simulink model "Model_simulink_no_Torque"  (R2017a)
settings: Solver=ode3  StartTime=0.0  StopTime=Tend  FixedStep=0.0006  RelTol=1e-3
values from neighbouring files (symbols this model uses):
  In = 130.7    [Skrypt_do_schematu.m]
  J = Js+Jmr    (= 5.82)    [Skrypt_do_schematu.m]
  Kp = 0.15*Un    (= 66)    [Skrypt_do_schematu.m]
  Kt = 10/(1.2*wn)    (= 0.0548810148593)    [Skrypt_do_schematu.m]
  Kw = J/(2*Kt*kz*Beta*psi)    [Skrypt_do_schematu.m]
  Lambda = 2    [Skrypt_do_schematu.m]
  m = T1    [Skrypt_do_schematu.m]
  Mn = psi * In    (= 350.156554572)    [Skrypt_do_schematu.m]
  psi = (Un-(Rt*In))/wn    (= 2.67908610996)    [Skrypt_do_schematu.m]
  Rt = 0.254    [Skrypt_do_schematu.m]
  T = Lt/Rt    (= 0.00641732283465)    [Skrypt_do_schematu.m]
  TR = 4*Beta    (= 0.16)    [Skrypt_do_schematu.m]
  Un = 440    [Skrypt_do_schematu.m]
  Uz0 = (Lambda*In)*((Y*B1)/(B1-Beta))    [Skrypt_do_schematu.m]
  V = (Beta*(Y*Kp*B))/((B1-Beta)*Rt)    [Skrypt_do_schematu.m]
  wn = (2*pi*n)/60    (= 151.843644924)    [Skrypt_do_schematu.m]
  Y = 7.8/(2.5*In)    (= 0.0238714613619)    [Skrypt_do_schematu.m]
settings Model: Creator=user  LastModifiedBy=a
settings DataIOCC: LimitDataPoints=on  SaveFormat=Array  SignalLoggingSaveFormat=ModelDataLogs
settings OptimizationCC: BlockReduction=off  BooleanDataType=off  ExpressionDepthLimit=2147483647  LifeSpan=inf
settings DebuggingCC: SaveWithParameterizedLinksMsg=none  UnderspecifiedInitializationDetection=Classic  MergeDetectMultiDrivingBlocksExec=none  SignalResolutionControl=TryResolveAllWithWarning  MultiTaskDSMMsg=warning  MultiTaskCondExecSysMsg=none  StateNameClashWarn=warning  SFUnexpectedBacktrackingDiag=warning  SFNoUnconditionalDefaultTransitionDiag=warning  SFExecutionAtInitializationDiag=none
settings HardwareCC: ProdBitPerPointer=32  ProdBitPerSizeT=32  ProdBitPerPtrDiffT=32  ProdLargestAtomicFloat=None  ProdIntDivRoundTo=Undefined  ProdEndianess=Unspecified  ProdWordSize=32  ProdHWDeviceType=32-bit Generic  TargetUnknown=on
settings ModelReferenceCC: PropagateSignalLabelsOutOfModel=off
settings GRTTargetCC: TargetLangStandard=C89/C90 (ANSI)  GeneratePreprocessorConditionals=Disable all
settings ConfigComp: CovMetricSettings=dw  CovHtmlReporting=on  CovSaveCumulativeToWorkspaceVar=on  CovSaveSingleToWorkspaceVar=on  CovExternalEMLEnable=off

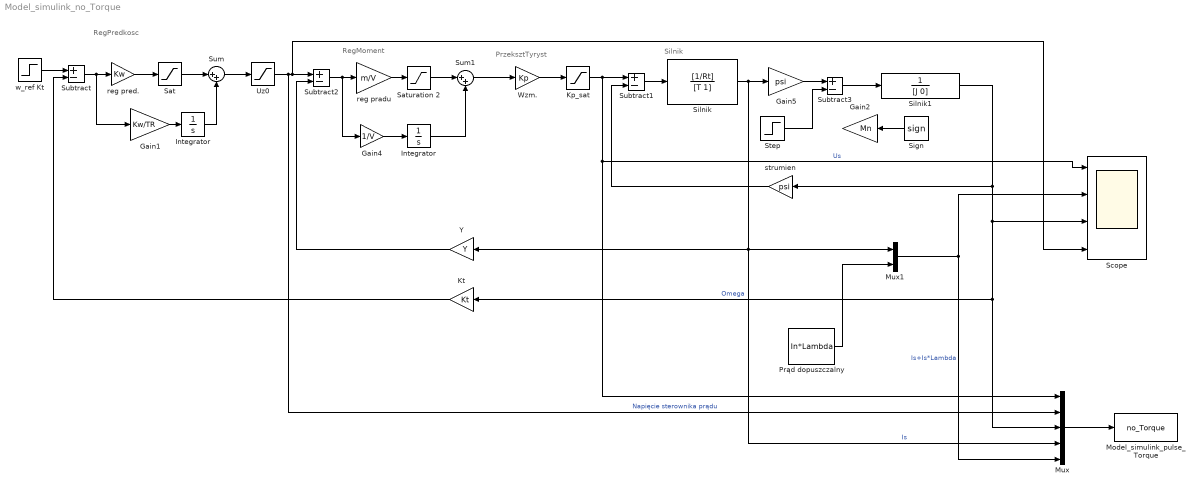
== system Model_simulink_no_Torque ==
  note: Silnik
  note: PrzeksztTyryst
  note: RegMoment
  note: RegPredkosc
  Gain1 : Gain  Gain=Kw/TR
  Gain2 : Gain  Gain=Mn
  Gain4 : Gain  Gain=1/V
  Gain5 : Gain  Gain=psi
  Integrator : Integrator  LimitOutput=on  UpperSaturationLimit=10  LowerSaturationLimit=-10
  "Integrator " : Integrator  LimitOutput=on  UpperSaturationLimit=10  LowerSaturationLimit=-10
  Kp_sat : Saturate  UpperLimit=1.5*Un  LowerLimit=-1.5*Un
  Kt : Gain  Gain=Kt
  Model_simulink_pulse_Torque : ToWorkspace  VariableName=no_Torque  SaveFormat=Structure With Time  SampleTime=-1
  Mux : Mux  Inputs=5
  Mux1 : Mux  Inputs=2
  Prąd dopuszczalny : Constant  Value=In*Lambda
  Sat : Saturate  UpperLimit=10  LowerLimit=-10
  Saturation 2 : Saturate  UpperLimit=10  LowerLimit=-10
  Scope : Scope  NumInputPorts=4
  Sign : Signum  ZeroCross=off
  Silnik : TransferFcn  Numerator=[1/Rt]  Denominator=[T 1]
  Silnik1 : TransferFcn  Numerator=1  Denominator=[J 0]
  Step : Step  Time=0  After=0  SampleTime=0
  Subtract{,1..3} (4 alike) : Sum  Inputs=+-
  Sum : Sum  Inputs=|++
  Sum1 : Sum  Inputs=|++
  Uz0 : Saturate  UpperLimit=Uz0  LowerLimit=-Uz0
  Wzm. : Gain  Gain=Kp
  Y : Gain  Gain=Y
  reg pradu : Gain  Gain=m/V
  reg pred. : Gain  Gain=Kw
  strumien : Gain  Gain=psi
  w_ref Kt : Step  Time=0  After=wn*Kt  SampleTime=0
  wires:
  w_ref Kt/1 -> Subtract/1
  Subtract/1 -> Gain1/1, reg pred./1
  Gain1/1 -> Integrator/1
  reg pradu/1 -> Saturation 2/1
  Wzm./1 -> Kp_sat/1
  Gain4/1 -> "Integrator "/1
  Subtract1/1 -> Silnik/1
  Silnik/1 -> Gain5/1, Mux/4, Y/1, Mux1/1  "Is"
  Gain5/1 -> Subtract3/1
  Subtract3/1 -> Silnik1/1
  strumien/1 -> Subtract1/2
  Kp_sat/1 -> Mux/1, Scope/1, Subtract1/1  "Us"
  Y/1 -> Subtract2/2
  Mux1/1 -> Mux/5, Scope/2  "Is+Is*Lambda"
  Prąd dopuszczalny/1 -> Mux1/2
  Uz0/1 -> Scope/4, Subtract2/1, Mux/2  "Napięcie sterownika prądu"
  Silnik1/1 -> Mux/3, Kt/1, Scope/3, strumien/1  "Omega"
  Kt/1 -> Subtract/2
  reg pred./1 -> Sat/1
  Saturation 2/1 -> Sum1/1
  Sum1/1 -> Wzm./1
  "Integrator "/1 -> Sum1/2
  Subtract2/1 -> Gain4/1, reg pradu/1
  Sat/1 -> Sum/1
  Sum/1 -> Uz0/1
  Integrator/1 -> Sum/2
  Mux/1 -> Model_simulink_pulse_Torque/1
  Sign/1 -> Gain2/1
  Step/1 -> Subtract3/2
